simulink model "plant"  (R2020a)
settings: Solver=VariableStepAuto  StartTime=0.0  StopTime=5  RelTol=1e-3
values from neighbouring files (symbols this model uses):
  A = [0, 1; 4.1*10^4, 0]    [kalman_params.m]
  B = [0; -9.12]    [kalman_params.m]
  C = [1 0;0 1]    [kalman_params.m]
  D = [0; 0]    [kalman_params.m]
undefined symbols (not defined in the file or in its folder): Kc
settings Model: Creator=prans  LastModifiedBy=prans

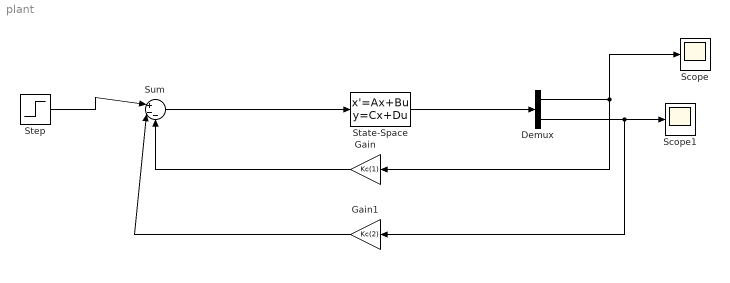
== system plant ==
  Demux : Demux  Outputs=2
  Gain : Gain  Gain=Kc(1)
  Gain1 : Gain  Gain=Kc(2)
  Scope : Scope
  Scope1 : Scope
  State-Space : StateSpace  A=A  B=B  C=C  D=D  InitialCondition=[1 0]
  Step : Step  Time=0  After=0  SampleTime=0
  Sum : Sum  Inputs=|+--
  wires:
  Step/1 -> Sum/1
  Demux/1 -> Scope/1, Gain/1
  Gain/1 -> Sum/3
  Gain1/1 -> Sum/2
  Demux/2 -> Scope1/1, Gain1/1
  Sum/1 -> State-Space/1
  State-Space/1 -> Demux/1
